simulink model "q13"  (R2021a)
settings: Solver=VariableStepAuto  StartTime=0.0  StopTime=100*1e-6  RelTol=1e-3
values from neighbouring files (symbols this model uses):
  cnst_sample_time = 1e-6*rig_samples_per_frame    (= 0.0001)    [q13_.m]
  erc_receive_delay = 10*log2(M)    [q13_.m]
  M = 4    [q13_.m]
  rig_sample_time = 1e-6    (= 1e-06)    [q13_.m]
  uc_dc_freq = 2.5e6    (= 2500000)    [q13_.m]
  uc_dc_sample_time = 1e-6/8    (= 1.25e-07)    [q13_.m]
libraries: commutil2 x2, dspsrcs4 x2, commdigbbndam3 x2, commfilt2 x2, commchan3 x1, commsink2 x1, commrandsrc3 x1
settings Model: Creator=Fatiha  LastModifiedBy=Fatiha

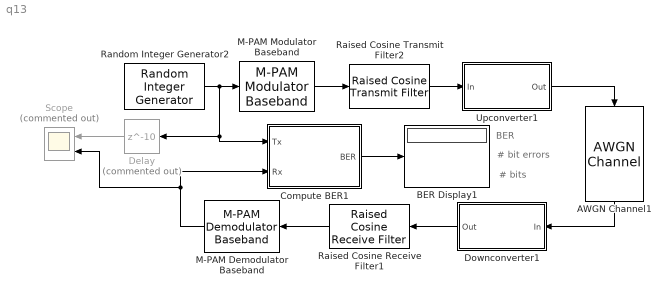
== system q13 ==
  note: # bits
  note: BER
  note: # bit errors
  AWGN Channel1 : commchan3/AWGN Channel  InputProcessing=Columns as channels (frame based)  seed=67  noiseMode="Signal to noise ratio  (Es/No)"  EbNodB=10  EsNodB=current_snr  SNRdB=10  bitsPerSym=1  Ps=awgn_input_signal_power  Tsym=awgn_symbol_period  variance=1
  BER Display1 : Display
  Compute BER1 : Subsystem
  Delay : Delay  Commented=on  DelayLength=10
  Downconverter1 : Subsystem
      mask Display: disp('Downconverter')
  M-PAM Demodulator Baseband : commdigbbndam3/M-PAM Demodulator Baseband  M=M  OutType=Integer  Dec=Gray  PowType=Average Power  MinDist=2  AvgPow=mod_demod_av_pow  PeakPow=1  outDtype1=Inherit via internal rule  outDtype2=Inherit via internal rule  denormFactorWordLen=16  denormFactorDataTypeStr=Inherit: Same word length as input  denormFactorLastDataTypeStr=Inherit: Same word length as input  prodOutWordLen=16  prodOutRoundingMode=Floor  prodOutOverflowMode=Wrap  prodOutOvFlMode=off  prodOutOvFlModeLastStrValue=off  sumWordLen=16
      settings: SourceProductBaseCode=CM
  M-PAM Modulator Baseband : commdigbbndam3/M-PAM Modulator Baseband  M=M  InType=Integer  Enc=Gray  PowType=Average Power  MinDist=2  AvgPow=mod_demod_av_pow  PeakPow=1  outDtype=double  outWordLen=16  outUDDataType=sfix(16)  outFracLenMode=Best precision  outFracLen=15  outDataTypeStr=double  outLastDataTypeStr=double
      settings: SourceProductBaseCode=CM
  Raised Cosine Receive Filter1 : commfilt2/Raised Cosine Receive Filter  filtType=Square root  R=0.2  filtSpan=10  N=8  downFactor=8  downOffset=0  filterGain=rcrf_gain  InputProcessing=Columns as channels (frame based)  RateOptions=Enforce single-rate processing  framing=Mute  checkCoeff=off  variableName=rcRxFilt1  currentFiltSpan=10  D=5  inputOffset=0  sampMode=Mute  saveAsFlag=0  rateMode=Downsampling  checkGain=Normalized  launchFVT=on  roundingMode=Floor  overflowMode=off  coeffDataTypeStr=Inherit: Same word length as input  coeffMin=[]  coeffMax=[]  coeffLastDataTypeStr=Inherit: Same word length as input  accumDataTypeStr=Inherit: Same as product output  accumLastDataTypeStr=Inherit: Same as product output  outputDataTypeStr=Inherit: Same as accumulator  outputMin=[]  outputMax=[]  outputLastDataTypeStr=Inherit: Same as accumulator
  Raised Cosine Transmit Filter2 : commfilt2/Raised Cosine Transmit Filter  filtType=Square root  R=0.2  filtSpan=10  N=8  filterGain=1  InputProcessing=Columns as channels (frame based)  RateOptions=Enforce single-rate processing  framing=Mute  checkCoeff=off  variableName=rcTxFilt2  checkGain=Normalized  sampMode=Mute  saveAsFlag=0  currentFiltSpan=10  D=5  launchFVT=on  roundingMode=Floor  overflowMode=off  coeffDataTypeStr=Inherit: Same word length as input  coeffMin=[]  coeffMax=[]  coeffLastDataTypeStr=Inherit: Same word length as input  outputDataTypeStr=Inherit: Same as accumulator  outputMin=[]  outputMax=[]  outputLastDataTypeStr=Inherit: Same as accumulator
  Random Integer Generator2 : commrandsrc3/Random Integer Generator  SetSize=M  SeedSource=Auto  Seed=0  SampleTime=rig_sample_time  SamplesPerFrame=rig_samples_per_frame  OutputDataType=double  SimulateUsing=Interpreted execution
  Scope : Scope  Commented=on  NumInputPorts=2
  Upconverter1 : Subsystem
      mask Display: disp('Upconverter')
  wires:
  Compute BER1/1(BER) -> BER Display1/1
  Random Integer Generator2/1 -> M-PAM Modulator Baseband/1, Delay/1, Compute BER1/1(Tx)
  M-PAM Modulator Baseband/1 -> Raised Cosine Transmit Filter2/1
  Downconverter1/1(Out) -> Raised Cosine Receive Filter1/1
  Upconverter1/1(Out) -> AWGN Channel1/1
  M-PAM Demodulator Baseband/1 -> Scope/2, Compute BER1/2(Rx)
  Raised Cosine Receive Filter1/1 -> M-PAM Demodulator Baseband/1
  AWGN Channel1/1 -> Downconverter1/1(In)
  Raised Cosine Transmit Filter2/1 -> Upconverter1/1(In)
  Delay/1 -> Scope/1

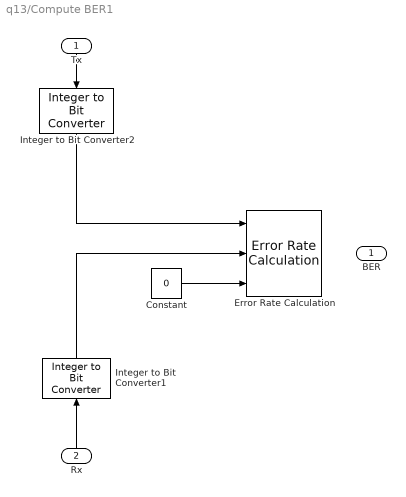
== system q13/Compute BER1 ==
  Tx : Inport
  Rx : Inport  Port=2
  Constant : Constant  Value=0  SampleTime=cnst_sample_time
  Error Rate Calculation : commsink2/Error Rate Calculation  N=erc_receive_delay  st_delay=0  cp_mode=Entire frame  subframe=[]  PMode=Workspace  WsName=ErrorVec  RsMode2=on  stop=off  numErr=100  maxBits=1e6
  Integer to Bit Converter1 : commutil2/Integer to Bit Converter  nbits=log2(M)  signedInputValues=Unsigned  bitOrder=LSB first  outDtype=boolean
  Integer to Bit Converter2 : commutil2/Integer to Bit Converter  nbits=log2(M)  signedInputValues=Unsigned  bitOrder=LSB first  outDtype=boolean
  BER : Outport  VectorParamsAs1DForOutWhenUnconnected=off
  wires:
  Integer to Bit Converter2/1 -> Error Rate Calculation/1
  Tx/1 -> Integer to Bit Converter2/1
  Rx/1 -> Integer to Bit Converter1/1
  Constant/1 -> Error Rate Calculation/3
  Integer to Bit Converter1/1 -> Error Rate Calculation/2
  ? -> BER/1

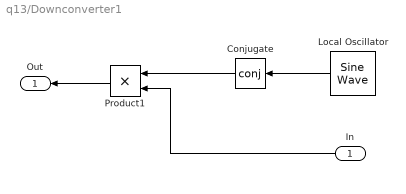
== system q13/Downconverter1 ==
  In : Inport
  Conjugate : Math  Operator=conj  SignedPower=on  SaturateOnIntegerOverflow=on
  Local Oscillator : dspsrcs4/Sine Wave  Amplitude=1  Frequency=uc_dc_freq  Phase=0  SampleMode=Discrete  OutComplex=Complex  CompMethod=Trigonometric fcn  TableSize=Speed  SampleTime=uc_dc_sample_time  SamplesPerFrame=uc_dc_samples_per_frame  ResetState=Restart at time zero  OutputFrames=off  dataType=double  wordLen=16  udDataType=sfix(16)  fracBitsMode=Best precision  numFracBits=15  OutDataTypeStr=double  LastOutDataTypeStr=double
  Product1 : Product  RndMeth=Zero
  Out : Outport  VectorParamsAs1DForOutWhenUnconnected=off
  wires:
  Conjugate/1 -> Product1/1
  Product1/1 -> Out/1
  In/1 -> Product1/2
  Local Oscillator/1 -> Conjugate/1

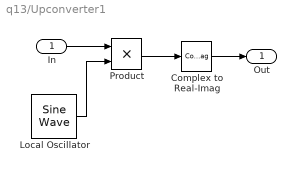
== system q13/Upconverter1 ==
  In : Inport
  Complex to Real-Imag : ComplexToRealImag  Output=Real
  Local Oscillator : dspsrcs4/Sine Wave  Amplitude=1  Frequency=uc_dc_freq  Phase=0  SampleMode=Discrete  OutComplex=Complex  CompMethod=Trigonometric fcn  TableSize=Speed  SampleTime=uc_dc_sample_time  SamplesPerFrame=uc_dc_samples_per_frame  ResetState=Restart at time zero  OutputFrames=off  dataType=double  wordLen=16  udDataType=sfix(16)  fracBitsMode=Best precision  numFracBits=15  OutDataTypeStr=double  LastOutDataTypeStr=double
  Product : Product  RndMeth=Zero
  Out : Outport  VectorParamsAs1DForOutWhenUnconnected=off
  wires:
  Complex to Real-Imag/1 -> Out/1
  Product/1 -> Complex to Real-Imag/1
  Local Oscillator/1 -> Product/2
  In/1 -> Product/1
